simulink model "velo_pi"  (R2025b)
settings: Solver=VariableStepAuto  StartTime=0.0  StopTime=10.0  RelTol=1e-3
libraries: arduino_io_lib x5
settings Model: Creator=nttha  LastModifiedBy=trong

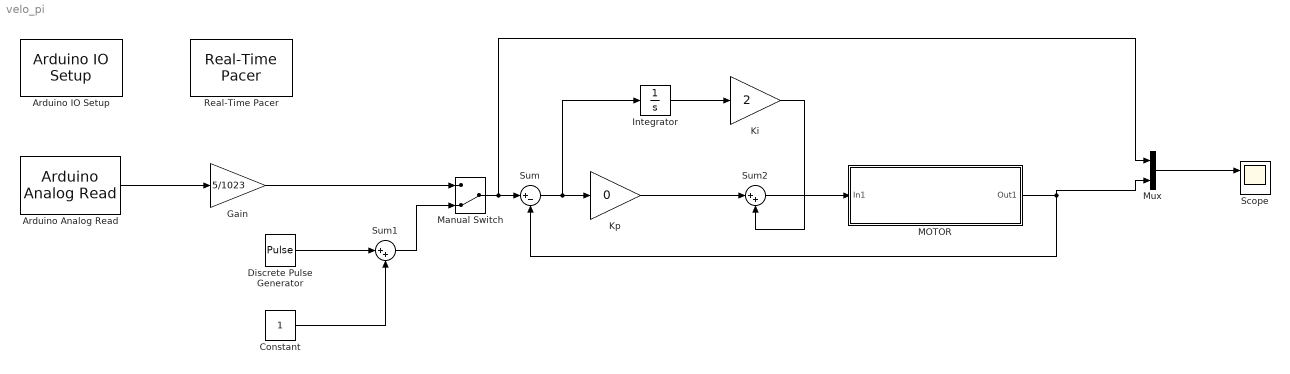
== system velo_pi ==
  Arduino Analog Read : arduino_io_lib/Arduino Analog Read  arduinoVar=Temporary arduino variable: Arduino1  arduinoPin=1  T=0.02
      settings: SourceProductName=Arduino IO Library
  Arduino IO Setup : arduino_io_lib/Arduino IO Setup  Priority=3  arduinoVar=Temporary arduino variable: Arduino1  workspaceVarName=a  comPort=COM3
      settings: SourceProductName=Arduino IO Library
  Constant : Constant
  Discrete Pulse Generator : DiscretePulseGenerator  Amplitude=0.5  Period=80  PulseWidth=40  SampleTime=1/20
  Gain : Gain  Gain=5/1023
  Integrator : Integrator
  Ki : Gain  Gain=2
  Kp : Gain  Gain=0
  MOTOR : Subsystem
  Manual Switch : ManualSwitch  CurrentSetting=0
  Mux : Mux  Inputs=2
  Real-Time Pacer : arduino_io_lib/Real-Time Pacer  simTimePerRealTime=1
      settings: SourceProductName=Arduino IO Library
  Scope : Scope  NumInputPorts=2
      settings: ActiveDisplayYMinimum=-1.4999999999999996  ActiveDisplayYMaximum=13.5
  Sum : Sum  Inputs=|+-
  Sum1 : Sum  Inputs=|++
  Sum2 : Sum  Inputs=|++
  wires:
  Arduino Analog Read/1 -> Gain/1
  MOTOR/1(Out1) -> Sum/2, Mux/2
  Mux/1 -> Scope/1
  Constant/1 -> Sum1/2
  Sum1/1 -> Manual Switch/2
  Gain/1 -> Manual Switch/1
  Sum/1 -> Integrator/1, Kp/1
  Manual Switch/1 -> Mux/1, Sum/1
  Discrete Pulse Generator/1 -> Sum1/1
  Integrator/1 -> Ki/1
  Kp/1 -> Sum2/1
  Sum2/1 -> MOTOR/1(In1)
  Ki/1 -> Sum2/2

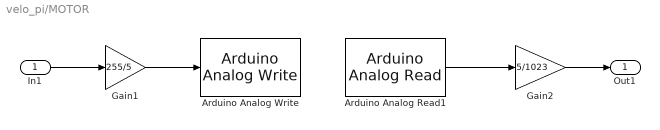
== system velo_pi/MOTOR ==
  In1 : Inport
  Arduino Analog Read1 : arduino_io_lib/Arduino Analog Read  arduinoVar=Temporary arduino variable: Arduino1  arduinoPin=0  T=0.02
      settings: SourceProductName=Arduino IO Library
  Arduino Analog Write : arduino_io_lib/Arduino Analog Write  arduinoVar=Temporary arduino variable: Arduino1  arduinoPin=3  T=0.02
      settings: SourceProductName=Arduino IO Library
  Gain1 : Gain  Gain=255/5
  Gain2 : Gain  Gain=5/1023
  Out1 : Outport
  wires:
  In1/1 -> Gain1/1
  Arduino Analog Read1/1 -> Gain2/1
  Gain1/1 -> Arduino Analog Write/1
  Gain2/1 -> Out1/1
